simulink model "exam2"  (R2021b)
settings: Solver=VariableStepAuto  StartTime=0.0  StopTime=10.0  RelTol=1e-3
libraries: mcbcontrolslib x1, simulink x1
settings Model: Creator=Mazen  LastModifiedBy=Mazen
settings DebuggingCC: UnconnectedInputMsg=none  UnconnectedOutputMsg=none  UnconnectedLineMsg=none
settings ModelReferenceCC: EnableRefExpFcnMdlSchedulingChecks=off
settings RTWCC: DLArmComputeVersion=20.02.1

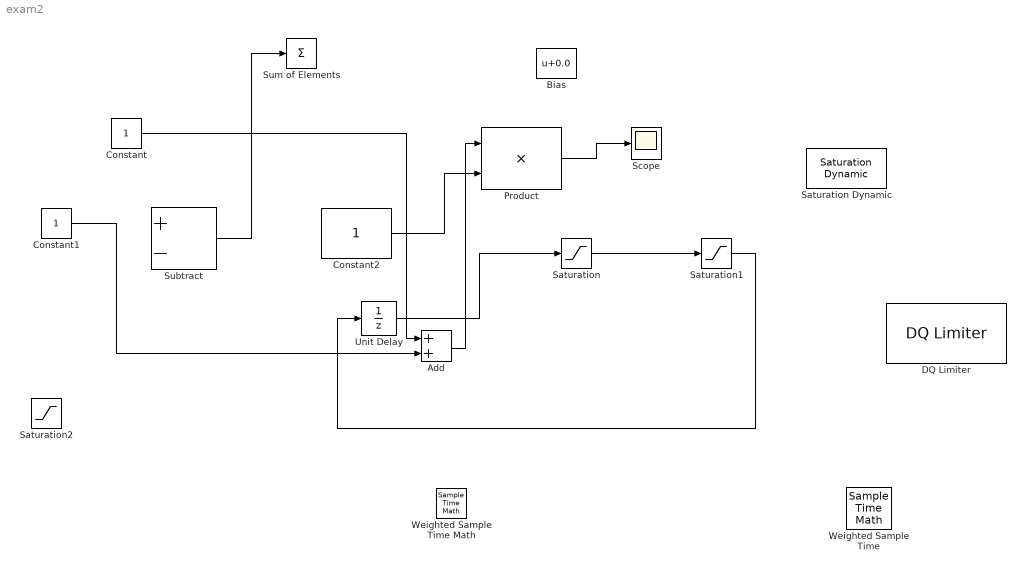
== system exam2 ==
  Add : Sum
  Bias : Bias  Bias=0.0
  Constant : Constant
  Constant1 : Constant
  Constant2 : Constant
  DQ Limiter : mcbcontrolslib/DQ Limiter  satMethodInputType=Specify via dialog  satMethodSelected=D-Q equivalence  satLimitInputType=Specify via dialog  Vmax=1
  Product : Product
  Saturation : Saturate
  Saturation Dynamic : simulink/Discontinuities/Saturation Dynamic  OutMin=[]  OutMax=[]  OutDataTypeStr=Inherit: Same as second input  OutDataType=fixdt(1, 16)  OutScaling=2^-10  DoSatur=off
  Saturation1 : Saturate
  Saturation2 : Saturate
  Scope : Scope
  Subtract : Sum  Inputs=+-
  Sum of Elements : Sum  Inputs=+
  Unit Delay : UnitDelay  SampleTime=-1  HasFrameUpgradeWarning=on
  Weighted Sample Time : SampleTimeMath  TsampMathOp=Ts Only
  Weighted Sample Time Math : SampleTimeMath
  wires:
  Constant1/1 -> Add/2
  Constant/1 -> Add/1
  Add/1 -> Product/1
  Constant2/1 -> Product/2
  Product/1 -> Scope/1
  Unit Delay/1 -> Saturation/1
  Saturation/1 -> Saturation1/1
  Saturation1/1 -> Unit Delay/1
  Subtract/1 -> Sum of Elements/1
